simulink model "koen_flux_observer_pll_model"  (R2024b)
settings: Solver=FixedStepDiscrete  StartTime=0.0  StopTime=0.05  FixedStep=6.25e-05  RelTol=1e-3
PreLoadFcn:
  | Ts=6.25e-05; Rs=0.53; Kp_pll=200; Ki_pll=10000; FOC_OBS_THETA_COMP_RAD=2.7239; omega_real=376.9911184; v_amp=6; i_amp=2;
undefined symbols (not defined in the file or in its folder): DiscIntNeverNeededParam
settings Model: Creator=10095  LastModifiedBy=10095

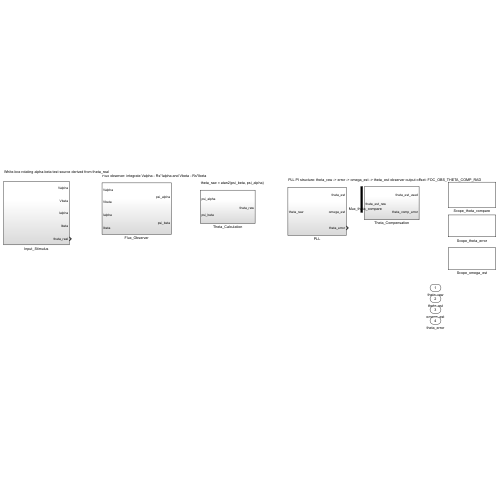
[thumbnail: Simulink's stored preview of the top-level diagram]
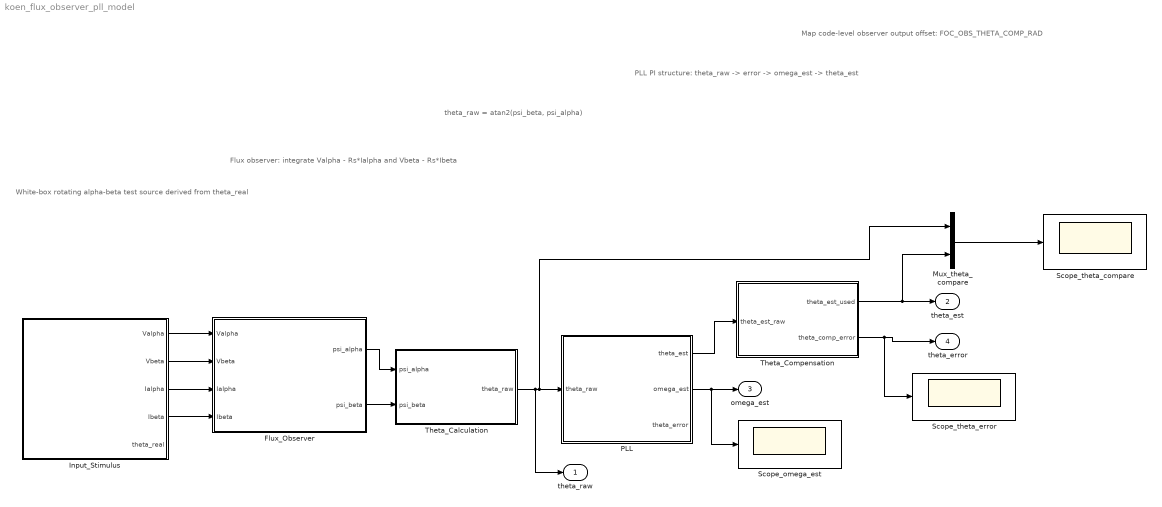
== system koen_flux_observer_pll_model ==
  note: White-box rotating alpha-beta test source derived from theta_real
  note: Flux observer: integrate Valpha - Rs*Ialpha and Vbeta - Rs*Ibeta
  note: theta_raw = atan2(psi_beta, psi_alpha)
  note: PLL PI structure: theta_raw -> error -> omega_est -> theta_est
  note: Map code-level observer output offset: FOC_OBS_THETA_COMP_RAD
  Flux_Observer : Subsystem  Description=Flux observer: integrate Valpha - Rs*Ialpha and Vbeta - Rs*Ibeta
  Input_Stimulus : Subsystem  Description=White-box rotating alpha-beta test source derived from theta_real
  Mux_theta_compare : Mux  Inputs=2
  PLL : Subsystem  Description=PLL PI structure: theta_raw -> error -> omega_est -> theta_est
  Scope_omega_est : Scope
  Scope_theta_compare : Scope
  Scope_theta_error : Scope
  Theta_Calculation : Subsystem  Description=theta_raw = atan2(psi_beta, psi_alpha)
  Theta_Compensation : Subsystem  Description=Map code-level observer output offset: FOC_OBS_THETA_COMP_RAD
  theta_raw : Outport
  theta_est : Outport  Port=2
  omega_est : Outport  Port=3
  theta_error : Outport  Port=4
  wires:
  PLL/1(theta_est) -> Theta_Compensation/1(theta_est_raw)
  PLL/2(omega_est) -> Scope_omega_est/1, omega_est/1
  Input_Stimulus/1(Valpha) -> Flux_Observer/1(Valpha)
  Input_Stimulus/4(Ibeta) -> Flux_Observer/4(Ibeta)
  Input_Stimulus/3(Ialpha) -> Flux_Observer/3(Ialpha)
  Theta_Compensation/1(theta_est_used) -> Mux_theta_compare/2, theta_est/1
  Input_Stimulus/2(Vbeta) -> Flux_Observer/2(Vbeta)
  Flux_Observer/2(psi_beta) -> Theta_Calculation/2(psi_beta)
  Flux_Observer/1(psi_alpha) -> Theta_Calculation/1(psi_alpha)
  Theta_Calculation/1(theta_raw) -> PLL/1(theta_raw), Mux_theta_compare/1, theta_raw/1
  Theta_Compensation/2(theta_comp_error) -> Scope_theta_error/1, theta_error/1
  Mux_theta_compare/1 -> Scope_theta_compare/1

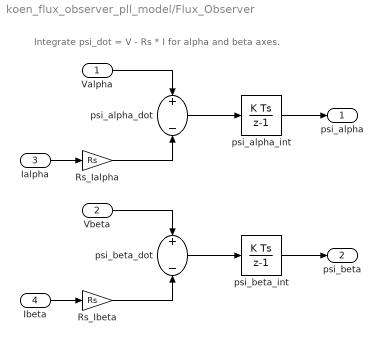
== system koen_flux_observer_pll_model/Flux_Observer ==
  note: Integrate psi_dot = V - Rs * I for alpha and beta axes.
  Valpha : Inport
  Vbeta : Inport  Port=2
  Ialpha : Inport  Port=3
  Ibeta : Inport  Port=4
  Rs_Ialpha : Gain  Gain=Rs
  Rs_Ibeta : Gain  Gain=Rs
  psi_alpha_dot : Sum  Inputs=+-
  psi_alpha_int : DiscreteIntegrator  SampleTime=Ts  ICPrevOutput=DiscIntNeverNeededParam  ICPrevScaledInput=DiscIntNeverNeededParam
  psi_beta_dot : Sum  Inputs=+-
  psi_beta_int : DiscreteIntegrator  SampleTime=Ts  ICPrevOutput=DiscIntNeverNeededParam  ICPrevScaledInput=DiscIntNeverNeededParam
  psi_alpha : Outport
  psi_beta : Outport  Port=2
  wires:
  Valpha/1 -> psi_alpha_dot/1
  Ibeta/1 -> Rs_Ibeta/1
  Ialpha/1 -> Rs_Ialpha/1
  Rs_Ialpha/1 -> psi_alpha_dot/2
  Vbeta/1 -> psi_beta_dot/1
  Rs_Ibeta/1 -> psi_beta_dot/2
  psi_alpha_dot/1 -> psi_alpha_int/1
  psi_beta_dot/1 -> psi_beta_int/1
  psi_alpha_int/1 -> psi_alpha/1
  psi_beta_int/1 -> psi_beta/1

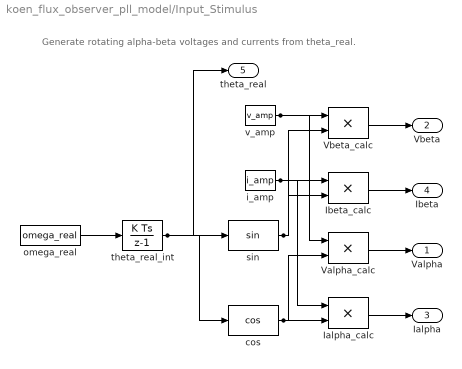
== system koen_flux_observer_pll_model/Input_Stimulus ==
  note: Generate rotating alpha-beta voltages and currents from theta_real.
  Ialpha_calc : Product
  Ibeta_calc : Product
  Valpha_calc : Product
  Vbeta_calc : Product
  cos : Trigonometry  Operator=cos
  i_amp : Constant  Value=i_amp
  omega_real : Constant  Value=omega_real
  sin : Trigonometry
  theta_real_int : DiscreteIntegrator  SampleTime=Ts  ICPrevOutput=DiscIntNeverNeededParam  ICPrevScaledInput=DiscIntNeverNeededParam
  v_amp : Constant  Value=v_amp
  Valpha : Outport
  Vbeta : Outport  Port=2
  Ialpha : Outport  Port=3
  Ibeta : Outport  Port=4
  theta_real : Outport  Port=5
  wires:
  omega_real/1 -> theta_real_int/1
  theta_real_int/1 -> cos/1, sin/1, theta_real/1
  cos/1 -> Valpha_calc/2, Ialpha_calc/2
  sin/1 -> Vbeta_calc/2, Ibeta_calc/2
  Valpha_calc/1 -> Valpha/1
  i_amp/1 -> Ialpha_calc/1, Ibeta_calc/1
  Vbeta_calc/1 -> Vbeta/1
  v_amp/1 -> Valpha_calc/1, Vbeta_calc/1
  Ialpha_calc/1 -> Ialpha/1
  Ibeta_calc/1 -> Ibeta/1

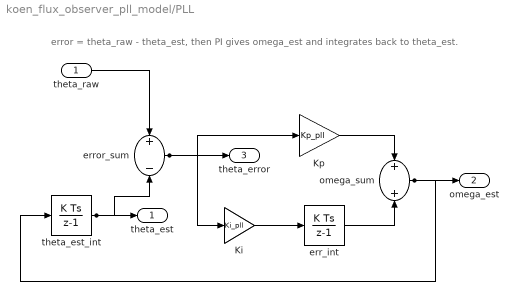
== system koen_flux_observer_pll_model/PLL ==
  note: error = theta_raw - theta_est, then PI gives omega_est and integrates back to theta_est.
  theta_raw : Inport
  Ki : Gain  Gain=Ki_pll
  Kp : Gain  Gain=Kp_pll
  err_int : DiscreteIntegrator  SampleTime=Ts  ICPrevOutput=DiscIntNeverNeededParam  ICPrevScaledInput=DiscIntNeverNeededParam
  error_sum : Sum  Inputs=+-
  omega_sum : Sum
  theta_est_int : DiscreteIntegrator  SampleTime=Ts  ICPrevOutput=DiscIntNeverNeededParam  ICPrevScaledInput=DiscIntNeverNeededParam
  theta_est : Outport
  omega_est : Outport  Port=2
  theta_error : Outport  Port=3
  wires:
  theta_raw/1 -> error_sum/1
  theta_est_int/1 -> error_sum/2, theta_est/1
  omega_sum/1 -> omega_est/1, theta_est_int/1
  err_int/1 -> omega_sum/2
  Kp/1 -> omega_sum/1
  Ki/1 -> err_int/1
  error_sum/1 -> theta_error/1, Ki/1, Kp/1

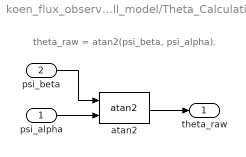
== system koen_flux_observer_pll_model/Theta_Calculation ==
  note: theta_raw = atan2(psi_beta, psi_alpha).
  psi_alpha : Inport
  psi_beta : Inport  Port=2
  atan2 : Trigonometry  Operator=atan2
  theta_raw : Outport
  wires:
  psi_alpha/1 -> atan2/2
  psi_beta/1 -> atan2/1
  atan2/1 -> theta_raw/1

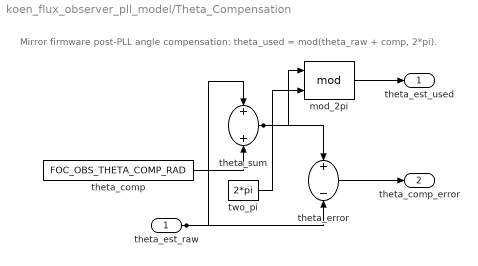
== system koen_flux_observer_pll_model/Theta_Compensation ==
  note: Mirror firmware post-PLL angle compensation: theta_used = mod(theta_raw + comp, 2*pi).
  theta_est_raw : Inport
  mod_2pi : Math  Operator=mod
  theta_comp : Constant  Value=FOC_OBS_THETA_COMP_RAD
  theta_error : Sum  Inputs=+-
  theta_sum : Sum
  two_pi : Constant  Value=2*pi
  theta_est_used : Outport
  theta_comp_error : Outport  Port=2
  wires:
  theta_est_raw/1 -> theta_sum/1, theta_error/2
  theta_comp/1 -> theta_sum/2
  theta_error/1 -> theta_comp_error/1
  mod_2pi/1 -> theta_est_used/1
  two_pi/1 -> mod_2pi/2
  theta_sum/1 -> theta_error/1, mod_2pi/1
